simulink model "Models_PID_FF"  (R2020a)
settings: Solver=FixedStepAuto  StartTime=0.0  StopTime=10  FixedStep=.01  MaxStep=.01  RelTol=1e-3
values from neighbouring files (symbols this model uses):
  c = app.cNmradsEditField.Value    [Feedforward_app_exported.m]
  g = 9.8    [Feedforward_app_exported.m]
  L = app.LmEditField.Value    [Feedforward_app_exported.m]
  m = app.massekgEditField.Value    [Feedforward_app_exported.m]
undefined symbols (not defined in the file or in its folder): Activate_FF
libraries: simulink_extras x3
settings Model: Creator=hussein  LastModifiedBy=hussein
settings DataIOCC: SaveOutput=off  SignalLogging=off  DSMLogging=off  ReturnWorkspaceOutputs=off

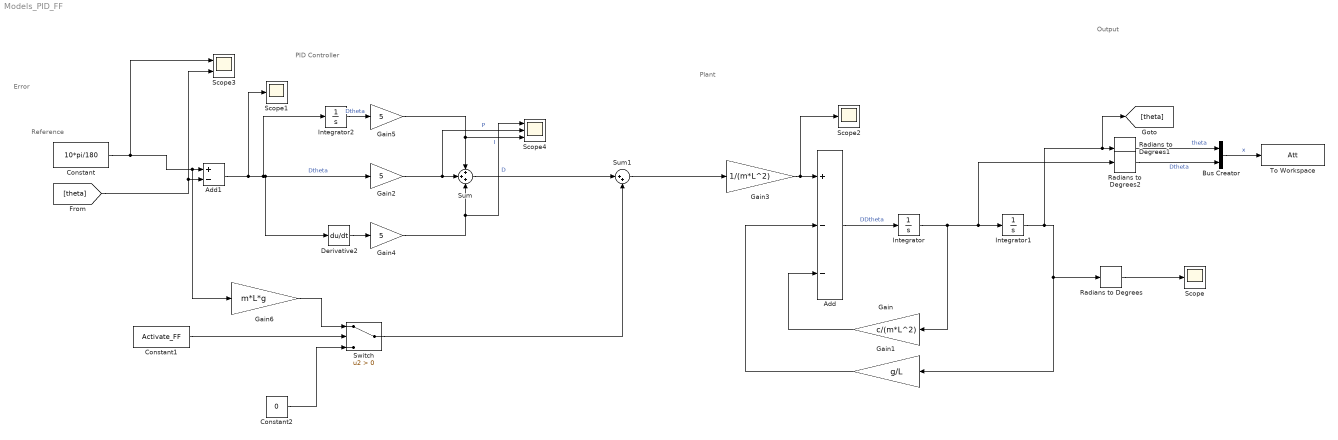
== system Models_PID_FF ==
  note: Output
  note: Plant
  note: Error
  note: Reference
  note: PID Controller
  Add : Sum  Inputs=+--
  Add1 : Sum  Inputs=+-
  Bus Creator : BusCreator  Inputs=2
  Constant : Constant  Value=10*pi/180
  Constant1 : Constant  Value=Activate_FF
  Constant2 : Constant  Value=0
  Derivative2 : Derivative
  Gain : Gain  Gain=c/(m*L^2)
  Gain1 : Gain  Gain=g/L
  Gain2 : Gain  Gain=5
  Gain3 : Gain  Gain=1/(m*L^2)
  Gain4 : Gain  Gain=5
  Gain5 : Gain  Gain=5
  Gain6 : Gain  Gain=m*L*g
  Integrator : Integrator
  Integrator1 : Integrator
  Integrator2 : Integrator
  Radians to Degrees : simulink_extras/Transformations/Radians to Degrees
  Radians to Degrees1 : simulink_extras/Transformations/Radians to Degrees
  Radians to Degrees2 : simulink_extras/Transformations/Radians to Degrees
  Scope : Scope
  Scope1 : Scope
  Scope2 : Scope
  Scope3 : Scope  NumInputPorts=2
  Scope4 : Scope  NumInputPorts=3
  Sum : Sum  Inputs=+++
  Sum1 : Sum  Inputs=|++
  Switch : Switch  Criteria=u2 > Threshold
  To Workspace : ToWorkspace  VariableName=Att  SaveFormat=Timeseries  SampleTime=-1
  wires:
  Add/1 -> Integrator/1  "DDtheta"
  Gain/1 -> Add/3
  Gain1/1 -> Add/2
  Gain3/1 -> Scope2/1, Add/1
  Bus Creator/1 -> To Workspace/1  "x"
  Add1/1 -> Integrator2/1, Derivative2/1, Gain2/1, Scope1/1  "Dtheta"
  Gain2/1 -> Scope4/2, Sum/2  "P"
  Gain5/1 -> Sum/1, Scope4/3  "I"
  Gain4/1 -> Scope4/1, Sum/3  "D"
  Radians to Degrees/1 -> Scope/1
  [theta] -> Scope3/2, Add1/2
  Sum/1 -> Sum1/1
  Integrator2/1 -> Gain5/1  "Dtheta"
  Derivative2/1 -> Gain4/1
  Constant1/1 -> Switch/2
  Constant2/1 -> Switch/3
  Constant/1 -> Scope3/1, Gain6/1, Add1/1
  Switch/1 -> Sum1/2
  Sum1/1 -> Gain3/1
  Gain6/1 -> Switch/1
  Integrator1/1 -> Radians to Degrees1/1, [theta], Gain1/1, Radians to Degrees/1
  Integrator/1 -> Gain/1, Radians to Degrees2/1, Integrator1/1
  Radians to Degrees1/1 -> Bus Creator/1  "theta"
  Radians to Degrees2/1 -> Bus Creator/2  "Dtheta"
